simulink library "Distribution_Lib"  (R2014a)
settings: Solver=ode45  StartTime=0.0  StopTime=10.0  RelTol=1e-3
libraries: powerlib x20, simulink x4, simulink_extras x4, Distribution_Lib x1
Description:
  | Copyright 2014 The MathWorks, Inc.
settings Model: Creator=smiller  LastModifiedBy=psanghvi

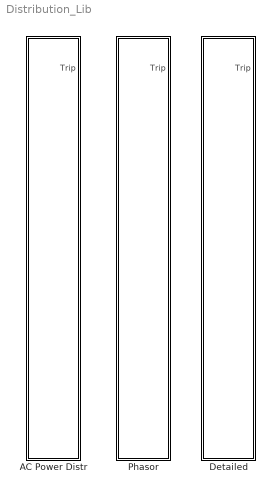
== system Distribution_Lib ==
  AC Power Distr : Subsystem  BlockChoice=Detailed
      settings: TemplateBlock=self  MemberBlocks=Detailed,Phasor
  Detailed : Subsystem  mask{FuseA=25, FuseB=200, FuseC=5, FuseD=30}
      mask prompts: FuseA "Breaker  TRU (Amps RMS)"; FuseB "Breaker AC motor (Amps RMS)"; FuseC "Breaker Lamp (Amps RMS)"; FuseD "Breaker Brushless (Amps RMS)"
  Phasor : Subsystem  mask{FuseA=25, FuseB=200, FuseC=5, FuseD=30}
      mask prompts: FuseA "Breaker  TRU (Amps RMS)"; FuseB "Breaker AC motor (Amps RMS)"; FuseC "Breaker Lamp (Amps RMS)"; FuseD "Breaker Brushless (Amps RMS)"

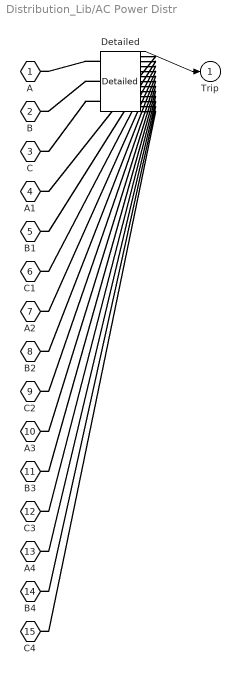
== system Distribution_Lib/AC Power Distr ==
  Detailed : Distribution_Lib/Detailed  FuseA=25  FuseB=200  FuseC=5  FuseD=30
  A : PMIOPort  Port=1  Side=Left
  B : PMIOPort  Port=2  Side=Left
  C : PMIOPort  Port=3  Side=Left
  A1 : PMIOPort  Port=4  Side=Right
  B1 : PMIOPort  Port=5  Side=Right
  C1 : PMIOPort  Port=6  Side=Right
  A2 : PMIOPort  Port=7  Side=Right
  B2 : PMIOPort  Port=8  Side=Right
  C2 : PMIOPort  Port=9  Side=Right
  A3 : PMIOPort  Port=10  Side=Right
  B3 : PMIOPort  Port=11  Side=Right
  C3 : PMIOPort  Port=12  Side=Right
  A4 : PMIOPort  Port=13  Side=Right
  B4 : PMIOPort  Port=14  Side=Right
  C4 : PMIOPort  Port=15  Side=Right
  Trip : Outport
  wires:
  Detailed/1 -> Trip/1
  connections:
  Detailed/LConn1 -- A/RConn1
  Detailed/LConn2 -- B/RConn1
  Detailed/LConn3 -- C/RConn1
  Detailed/RConn1 -- A1/RConn1
  Detailed/RConn2 -- B1/RConn1
  Detailed/RConn3 -- C1/RConn1
  Detailed/RConn4 -- A2/RConn1
  Detailed/RConn5 -- B2/RConn1
  Detailed/RConn6 -- C2/RConn1
  Detailed/RConn7 -- A3/RConn1
  Detailed/RConn8 -- B3/RConn1
  Detailed/RConn9 -- C3/RConn1
  Detailed/RConn10 -- A4/RConn1
  Detailed/RConn11 -- B4/RConn1
  Detailed/RConn12 -- C4/RConn1

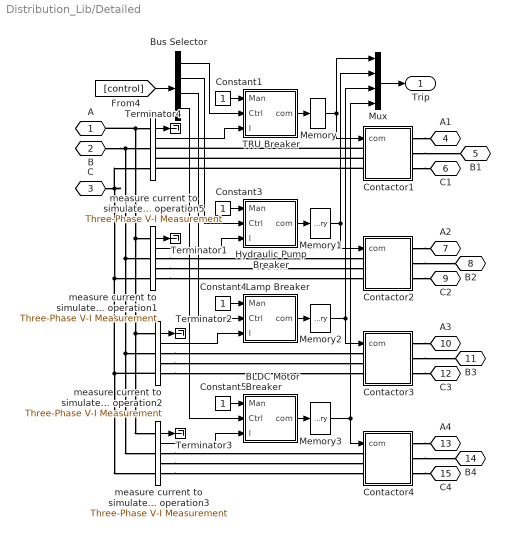
== system Distribution_Lib/Detailed ==
  BLDC Motor Breaker : Subsystem
  Bus Selector : BusSelector  OutputSignals=TRU_B,AC_Pump_B,AC_Lamp_B,AC_BLDC_B
  Constant{1,3..5} (4 alike) : Constant  OutDataTypeStr=boolean
  Contactor1 : Subsystem
  Contactor2 : Subsystem
  Contactor3 : Subsystem
  Contactor4 : Subsystem
  Hydraulic Pump Breaker : Subsystem
  Lamp Breaker : Subsystem
  Memory{,1..3} (4 alike) : Memory  X0=1
  Mux : Mux
  TRU Breaker : Subsystem
  Terminator{1..4} (4 alike) : Terminator
  measure current to simulate fuse operation{1..3,5} (4 alike) : powerlib/Measurements/Three-Phase V-I Measurement  VoltageMeasurement=phase-to-ground  SetLabelV=off  LabelV=Vabc  Vpu=off  VpuLL=off  CurrentMeasurement=yes  SetLabelI=off  LabelI=Iabc  Ipu=off  Pbase=100e6  Vbase=500e3  OutputType=Complex  PhasorSimulation=on  PSBequivalent=0
  A : PMIOPort  Port=1  Side=Left
  B : PMIOPort  Port=2  Side=Left
  C : PMIOPort  Port=3  Side=Left
  A1 : PMIOPort  Port=4  Side=Right
  B1 : PMIOPort  Port=5  Side=Right
  C1 : PMIOPort  Port=6  Side=Right
  A2 : PMIOPort  Port=7  Side=Right
  B2 : PMIOPort  Port=8  Side=Right
  C2 : PMIOPort  Port=9  Side=Right
  A3 : PMIOPort  Port=10  Side=Right
  B3 : PMIOPort  Port=11  Side=Right
  C3 : PMIOPort  Port=12  Side=Right
  A4 : PMIOPort  Port=13  Side=Right
  B4 : PMIOPort  Port=14  Side=Right
  C4 : PMIOPort  Port=15  Side=Right
  Trip : Outport
  wires:
  Memory/1 -> Contactor1/1(com), Mux/1
  Bus Selector/4 -> BLDC Motor Breaker/2(Ctrl)
  Bus Selector/3 -> Lamp Breaker/2(Ctrl)
  Bus Selector/2 -> Hydraulic Pump Breaker/2(Ctrl)
  [control] -> Bus Selector/1
  BLDC Motor Breaker/1(com) -> Memory3/1
  measure current to simulate fuse operation3/2 -> BLDC Motor Breaker/3(I)
  Constant5/1 -> BLDC Motor Breaker/1(Man)
  Constant4/1 -> Lamp Breaker/1(Man)
  Hydraulic Pump Breaker/1(com) -> Memory1/1
  Constant3/1 -> Hydraulic Pump Breaker/1(Man)
  Bus Selector/1 -> TRU Breaker/2(Ctrl)
  Memory1/1 -> Mux/2, Contactor2/1(com)
  measure current to simulate fuse operation5/2 -> TRU Breaker/3(I)
  TRU Breaker/1(com) -> Memory/1
  measure current to simulate fuse operation1/2 -> Hydraulic Pump Breaker/3(I)
  measure current to simulate fuse operation2/2 -> Lamp Breaker/3(I)
  Lamp Breaker/1(com) -> Memory2/1
  Mux/1 -> Trip/1
  Memory2/1 -> Mux/3, Contactor3/1(com)
  Memory3/1 -> Mux/4, Contactor4/1(com)
  Constant1/1 -> TRU Breaker/1(Man)
  measure current to simulate fuse operation2/1 -> Terminator2/1
  measure current to simulate fuse operation3/1 -> Terminator3/1
  measure current to simulate fuse operation1/1 -> Terminator1/1
  measure current to simulate fuse operation5/1 -> Terminator4/1
  connections:
  Contactor1/RConn2 -- B1/RConn1
  Contactor1/LConn3 -- measure current to simulate fuse operation5/RConn3
  Contactor1/LConn1 -- measure current to simulate fuse operation5/RConn1
  Contactor1/RConn3 -- C1/RConn1
  Contactor1/RConn1 -- A1/RConn1
  Contactor1/LConn2 -- measure current to simulate fuse operation5/RConn2
  measure current to simulate fuse operation1/LConn1 -- measure current to simulate fuse operation3/LConn1 -- measure current to simulate fuse operation2/LConn1 -- A/RConn1 -- measure current to simulate fuse operation5/LConn1
  measure current to simulate fuse operation1/LConn2 -- B/RConn1 -- measure current to simulate fuse operation5/LConn2 -- measure current to simulate fuse operation3/LConn2 -- measure current to simulate fuse operation2/LConn2
  measure current to simulate fuse operation1/LConn3 -- measure current to simulate fuse operation3/LConn3 -- measure current to simulate fuse operation2/LConn3 -- measure current to simulate fuse operation5/LConn3 -- C/RConn1
  measure current to simulate fuse operation1/RConn1 -- Contactor2/LConn1
  Contactor2/RConn2 -- B2/RConn1
  measure current to simulate fuse operation1/RConn3 -- Contactor2/LConn3
  Contactor3/RConn1 -- A3/RConn1
  measure current to simulate fuse operation2/RConn2 -- Contactor3/LConn2
  measure current to simulate fuse operation2/RConn3 -- Contactor3/LConn3
  measure current to simulate fuse operation3/RConn1 -- Contactor4/LConn1
  measure current to simulate fuse operation3/RConn2 -- Contactor4/LConn2
  measure current to simulate fuse operation3/RConn3 -- Contactor4/LConn3
  Contactor2/RConn1 -- A2/RConn1
  Contactor3/RConn2 -- B3/RConn1
  measure current to simulate fuse operation1/RConn2 -- Contactor2/LConn2
  Contactor2/RConn3 -- C2/RConn1
  Contactor4/RConn3 -- C4/RConn1
  Contactor4/RConn1 -- A4/RConn1
  Contactor3/RConn3 -- C3/RConn1
  measure current to simulate fuse operation2/RConn1 -- Contactor3/LConn1
  Contactor4/RConn2 -- B4/RConn1

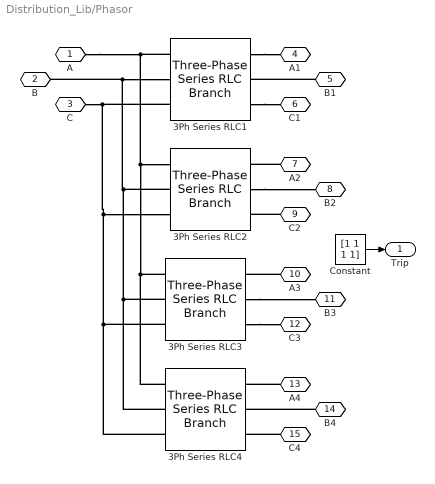
== system Distribution_Lib/Phasor ==
  3Ph Series RLC{1..4} (4 alike) : powerlib/Elements/Three-Phase Series RLC Branch  LConnTagsString=A|B|C  RConnTagsString=A|B|C  BranchType=R  Resistance=1e-3  Inductance=1e-3  Capacitance=1e-6  Measurements=None
  Constant : Constant  Value=[1 1 1 1]
  A : PMIOPort  Port=1  Side=Left
  B : PMIOPort  Port=2  Side=Left
  C : PMIOPort  Port=3  Side=Left
  A1 : PMIOPort  Port=4  Side=Right
  B1 : PMIOPort  Port=5  Side=Right
  C1 : PMIOPort  Port=6  Side=Right
  A2 : PMIOPort  Port=7  Side=Right
  B2 : PMIOPort  Port=8  Side=Right
  C2 : PMIOPort  Port=9  Side=Right
  A3 : PMIOPort  Port=10  Side=Right
  B3 : PMIOPort  Port=11  Side=Right
  C3 : PMIOPort  Port=12  Side=Right
  A4 : PMIOPort  Port=13  Side=Right
  B4 : PMIOPort  Port=14  Side=Right
  C4 : PMIOPort  Port=15  Side=Right
  Trip : Outport
  wires:
  Constant/1 -> Trip/1
  connections:
  C/RConn1 -- 3Ph Series RLC4/LConn3 -- 3Ph Series RLC3/LConn3 -- 3Ph Series RLC2/LConn3 -- 3Ph Series RLC1/LConn3
  A/RConn1 -- 3Ph Series RLC4/LConn1 -- 3Ph Series RLC3/LConn1 -- 3Ph Series RLC2/LConn1 -- 3Ph Series RLC1/LConn1
  B/RConn1 -- 3Ph Series RLC4/LConn2 -- 3Ph Series RLC3/LConn2 -- 3Ph Series RLC2/LConn2 -- 3Ph Series RLC1/LConn2
  3Ph Series RLC1/RConn1 -- A1/RConn1
  B1/RConn1 -- 3Ph Series RLC1/RConn2
  3Ph Series RLC1/RConn3 -- C1/RConn1
  A2/RConn1 -- 3Ph Series RLC2/RConn1
  3Ph Series RLC2/RConn2 -- B2/RConn1
  C2/RConn1 -- 3Ph Series RLC2/RConn3
  A3/RConn1 -- 3Ph Series RLC3/RConn1
  3Ph Series RLC3/RConn2 -- B3/RConn1
  3Ph Series RLC3/RConn3 -- C3/RConn1
  A4/RConn1 -- 3Ph Series RLC4/RConn1
  B4/RConn1 -- 3Ph Series RLC4/RConn2
  C4/RConn1 -- 3Ph Series RLC4/RConn3

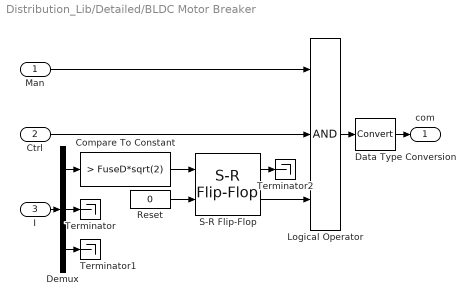
== system Distribution_Lib/Detailed/BLDC Motor Breaker ==
  Man : Inport
  Ctrl : Inport  Port=2
  I : Inport  Port=3
  Compare To Constant : simulink/Logic and Bit Operations/Compare To Constant  relop=>  const=FuseD*sqrt(2)  OutDataTypeStr=boolean  ZeroCross=off
  Data Type Conversion : DataTypeConversion
  Demux : Demux  Outputs=3
  Logical Operator : Logic  Inputs=3  AllPortsSameDT=off  OutDataTypeStr=boolean
  Reset : Constant  Value=0  OutDataTypeStr=boolean
  S-R Flip-Flop : simulink_extras/Flip Flops/S-R Flip-Flop  initial_condition=0
  Terminator : Terminator
  Terminator1 : Terminator
  Terminator2 : Terminator
  com : Outport
  wires:
  Ctrl/1 -> Logical Operator/2
  S-R Flip-Flop/2 -> Logical Operator/3
  I/1 -> Demux/1
  Demux/1 -> Compare To Constant/1
  Logical Operator/1 -> Data Type Conversion/1
  Man/1 -> Logical Operator/1
  Data Type Conversion/1 -> com/1
  Compare To Constant/1 -> S-R Flip-Flop/1
  Demux/2 -> Terminator/1
  Demux/3 -> Terminator1/1
  Reset/1 -> S-R Flip-Flop/2
  S-R Flip-Flop/1 -> Terminator2/1

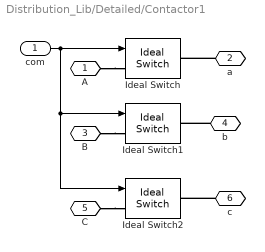
== system Distribution_Lib/Detailed/Contactor1 ==
  com : Inport
  Ideal Switch : powerlib/Power Electronics/Ideal Switch  Ron=0.001  Lon=0  IC=0  Rs=1e3  Cs=inf  Measurements=off
  Ideal Switch1 : powerlib/Power Electronics/Ideal Switch  Ron=0.001  Lon=0  IC=0  Rs=1e3  Cs=inf  Measurements=off
  Ideal Switch2 : powerlib/Power Electronics/Ideal Switch  Ron=0.001  Lon=0  IC=0  Rs=1e3  Cs=inf  Measurements=off
  A : PMIOPort  Port=1  Side=Left
  a : PMIOPort  Port=2  Side=Right
  B : PMIOPort  Port=3  Side=Left
  b : PMIOPort  Port=4  Side=Right
  C : PMIOPort  Port=5  Side=Left
  c : PMIOPort  Port=6  Side=Right
  wires:
  com/1 -> Ideal Switch1/1, Ideal Switch2/1, Ideal Switch/1
  connections:
  c/RConn1 -- Ideal Switch2/RConn1
  C/RConn1 -- Ideal Switch2/LConn1
  b/RConn1 -- Ideal Switch1/RConn1
  B/RConn1 -- Ideal Switch1/LConn1
  a/RConn1 -- Ideal Switch/RConn1
  A/RConn1 -- Ideal Switch/LConn1

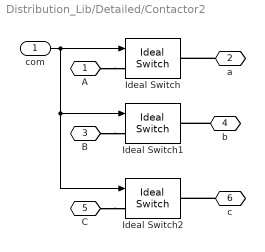
== system Distribution_Lib/Detailed/Contactor2 ==
  com : Inport
  Ideal Switch : powerlib/Power Electronics/Ideal Switch  Ron=0.001  Lon=0  IC=0  Rs=1e3  Cs=inf  Measurements=off
  Ideal Switch1 : powerlib/Power Electronics/Ideal Switch  Ron=0.001  Lon=0  IC=0  Rs=1e3  Cs=inf  Measurements=off
  Ideal Switch2 : powerlib/Power Electronics/Ideal Switch  Ron=0.001  Lon=0  IC=0  Rs=1e3  Cs=inf  Measurements=off
  A : PMIOPort  Port=1  Side=Left
  a : PMIOPort  Port=2  Side=Right
  B : PMIOPort  Port=3  Side=Left
  b : PMIOPort  Port=4  Side=Right
  C : PMIOPort  Port=5  Side=Left
  c : PMIOPort  Port=6  Side=Right
  wires:
  com/1 -> Ideal Switch/1, Ideal Switch2/1, Ideal Switch1/1
  connections:
  A/RConn1 -- Ideal Switch/LConn1
  a/RConn1 -- Ideal Switch/RConn1
  B/RConn1 -- Ideal Switch1/LConn1
  b/RConn1 -- Ideal Switch1/RConn1
  C/RConn1 -- Ideal Switch2/LConn1
  c/RConn1 -- Ideal Switch2/RConn1

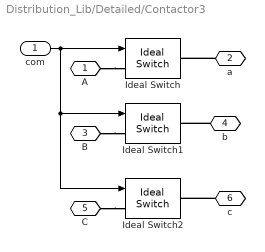
== system Distribution_Lib/Detailed/Contactor3 ==
  com : Inport
  Ideal Switch : powerlib/Power Electronics/Ideal Switch  Ron=0.001  Lon=0  IC=0  Rs=1e3  Cs=inf  Measurements=off
  Ideal Switch1 : powerlib/Power Electronics/Ideal Switch  Ron=0.001  Lon=0  IC=0  Rs=1e3  Cs=inf  Measurements=off
  Ideal Switch2 : powerlib/Power Electronics/Ideal Switch  Ron=0.001  Lon=0  IC=0  Rs=1e3  Cs=inf  Measurements=off
  A : PMIOPort  Port=1  Side=Left
  a : PMIOPort  Port=2  Side=Right
  B : PMIOPort  Port=3  Side=Left
  b : PMIOPort  Port=4  Side=Right
  C : PMIOPort  Port=5  Side=Left
  c : PMIOPort  Port=6  Side=Right
  wires:
  com/1 -> Ideal Switch1/1, Ideal Switch2/1, Ideal Switch/1
  connections:
  c/RConn1 -- Ideal Switch2/RConn1
  C/RConn1 -- Ideal Switch2/LConn1
  b/RConn1 -- Ideal Switch1/RConn1
  B/RConn1 -- Ideal Switch1/LConn1
  a/RConn1 -- Ideal Switch/RConn1
  A/RConn1 -- Ideal Switch/LConn1

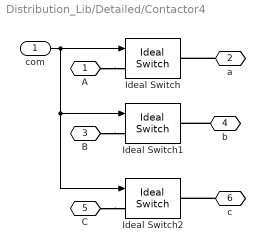
== system Distribution_Lib/Detailed/Contactor4 ==
  com : Inport
  Ideal Switch : powerlib/Power Electronics/Ideal Switch  Ron=0.001  Lon=0  IC=0  Rs=1e3  Cs=inf  Measurements=off
  Ideal Switch1 : powerlib/Power Electronics/Ideal Switch  Ron=0.001  Lon=0  IC=0  Rs=1e3  Cs=inf  Measurements=off
  Ideal Switch2 : powerlib/Power Electronics/Ideal Switch  Ron=0.001  Lon=0  IC=0  Rs=1e3  Cs=inf  Measurements=off
  A : PMIOPort  Port=1  Side=Left
  a : PMIOPort  Port=2  Side=Right
  B : PMIOPort  Port=3  Side=Left
  b : PMIOPort  Port=4  Side=Right
  C : PMIOPort  Port=5  Side=Left
  c : PMIOPort  Port=6  Side=Right
  wires:
  com/1 -> Ideal Switch/1, Ideal Switch2/1, Ideal Switch1/1
  connections:
  A/RConn1 -- Ideal Switch/LConn1
  a/RConn1 -- Ideal Switch/RConn1
  B/RConn1 -- Ideal Switch1/LConn1
  b/RConn1 -- Ideal Switch1/RConn1
  C/RConn1 -- Ideal Switch2/LConn1
  c/RConn1 -- Ideal Switch2/RConn1

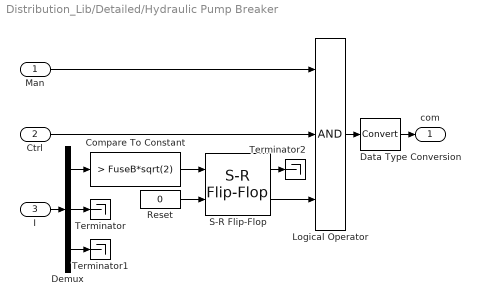
== system Distribution_Lib/Detailed/Hydraulic Pump Breaker ==
  Man : Inport
  Ctrl : Inport  Port=2
  I : Inport  Port=3
  Compare To Constant : simulink/Logic and Bit Operations/Compare To Constant  relop=>  const=FuseB*sqrt(2)  OutDataTypeStr=boolean  ZeroCross=off
  Data Type Conversion : DataTypeConversion
  Demux : Demux  Outputs=3
  Logical Operator : Logic  Inputs=3  AllPortsSameDT=off  OutDataTypeStr=boolean
  Reset : Constant  Value=0  OutDataTypeStr=boolean
  S-R Flip-Flop : simulink_extras/Flip Flops/S-R Flip-Flop  initial_condition=0
  Terminator : Terminator
  Terminator1 : Terminator
  Terminator2 : Terminator
  com : Outport
  wires:
  Ctrl/1 -> Logical Operator/2
  S-R Flip-Flop/2 -> Logical Operator/3
  I/1 -> Demux/1
  Demux/1 -> Compare To Constant/1
  Logical Operator/1 -> Data Type Conversion/1
  Man/1 -> Logical Operator/1
  Data Type Conversion/1 -> com/1
  Compare To Constant/1 -> S-R Flip-Flop/1
  Demux/2 -> Terminator/1
  Demux/3 -> Terminator1/1
  Reset/1 -> S-R Flip-Flop/2
  S-R Flip-Flop/1 -> Terminator2/1

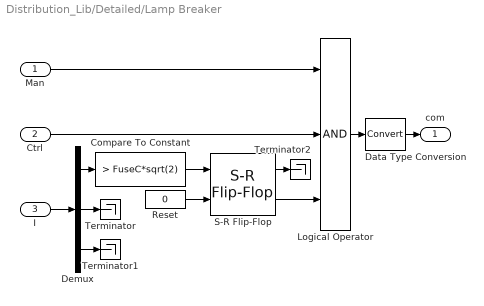
== system Distribution_Lib/Detailed/Lamp Breaker ==
  Man : Inport
  Ctrl : Inport  Port=2
  I : Inport  Port=3
  Compare To Constant : simulink/Logic and Bit Operations/Compare To Constant  relop=>  const=FuseC*sqrt(2)  OutDataTypeStr=boolean  ZeroCross=off
  Data Type Conversion : DataTypeConversion
  Demux : Demux  Outputs=3
  Logical Operator : Logic  Inputs=3  AllPortsSameDT=off  OutDataTypeStr=boolean
  Reset : Constant  Value=0  OutDataTypeStr=boolean
  S-R Flip-Flop : simulink_extras/Flip Flops/S-R Flip-Flop  initial_condition=0
  Terminator : Terminator
  Terminator1 : Terminator
  Terminator2 : Terminator
  com : Outport
  wires:
  Ctrl/1 -> Logical Operator/2
  S-R Flip-Flop/2 -> Logical Operator/3
  I/1 -> Demux/1
  Demux/1 -> Compare To Constant/1
  Logical Operator/1 -> Data Type Conversion/1
  Man/1 -> Logical Operator/1
  Data Type Conversion/1 -> com/1
  Compare To Constant/1 -> S-R Flip-Flop/1
  Demux/2 -> Terminator/1
  Demux/3 -> Terminator1/1
  Reset/1 -> S-R Flip-Flop/2
  S-R Flip-Flop/1 -> Terminator2/1

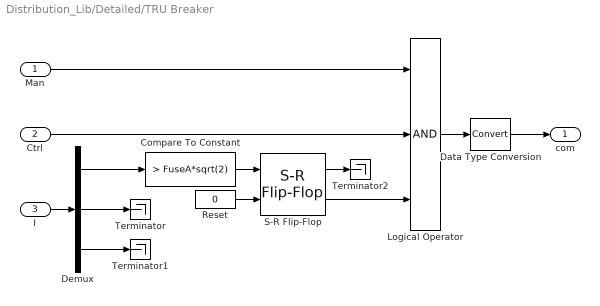
== system Distribution_Lib/Detailed/TRU Breaker ==
  Man : Inport
  Ctrl : Inport  Port=2
  I : Inport  Port=3
  Compare To Constant : simulink/Logic and Bit Operations/Compare To Constant  relop=>  const=FuseA*sqrt(2)  OutDataTypeStr=boolean  ZeroCross=off
  Data Type Conversion : DataTypeConversion
  Demux : Demux  Outputs=3
  Logical Operator : Logic  Inputs=3  AllPortsSameDT=off  OutDataTypeStr=boolean
  Reset : Constant  Value=0  OutDataTypeStr=boolean
  S-R Flip-Flop : simulink_extras/Flip Flops/S-R Flip-Flop  initial_condition=0
  Terminator : Terminator
  Terminator1 : Terminator
  Terminator2 : Terminator
  com : Outport
  wires:
  Ctrl/1 -> Logical Operator/2
  S-R Flip-Flop/2 -> Logical Operator/3
  I/1 -> Demux/1
  Demux/1 -> Compare To Constant/1
  Logical Operator/1 -> Data Type Conversion/1
  Man/1 -> Logical Operator/1
  Data Type Conversion/1 -> com/1
  Compare To Constant/1 -> S-R Flip-Flop/1
  Demux/2 -> Terminator/1
  Demux/3 -> Terminator1/1
  Reset/1 -> S-R Flip-Flop/2
  S-R Flip-Flop/1 -> Terminator2/1
